simulink model "simulacao_sem_linearizar_prbs2"  (R2017a)
settings: Solver=VariableStepAuto  StartTime=0.0  StopTime=100  RelTol=1e-3
values from neighbouring files (symbols this model uses):
  a = -9128    [prepare_y_prbs.m]
undefined symbols (not defined in the file or in its folder): g, m
libraries: simulink x1
settings Model: Creator=Mateus  LastModifiedBy=Vicente

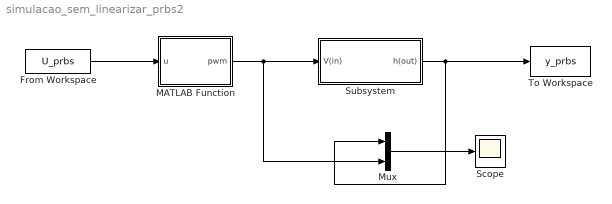
== system simulacao_sem_linearizar_prbs2 ==
  From Workspace : FromWorkspace  VariableName=U_prbs  SampleTime=0.05  Interpolate=off  OutputAfterFinalValue=Setting to zero
  MATLAB Function : MATLAB Function  TreatAsAtomicUnit=on
  Mux : Mux  Inputs=2
  Scope : Scope
  Subsystem : Subsystem
  To Workspace : ToWorkspace  VariableName=y_prbs  SaveFormat=Timeseries  SampleTime=0.05
  wires:
  From Workspace/1 -> MATLAB Function/1(u)
  MATLAB Function/1(pwm) -> Mux/2, Subsystem/1(V(in))
  Subsystem/1(h(out)) -> Mux/1, To Workspace/1
  Mux/1 -> Scope/1

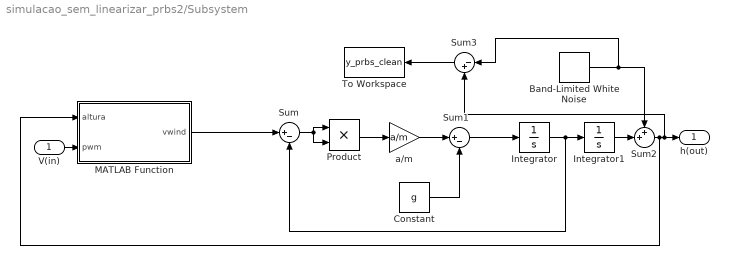
== system simulacao_sem_linearizar_prbs2/Subsystem ==
  V(in) : Inport
  Band-Limited White Noise : simulink/Sources/Band-Limited White Noise  Cov=[0.02]  Ts=0.1  seed=[23341]
  Constant : Constant  Value=g
  Integrator : Integrator
  Integrator1 : Integrator  InitialCondition=30
  MATLAB Function : MATLAB Function  TreatAsAtomicUnit=on
  Product : Product
  Sum : Sum  Inputs=|+-
  Sum1 : Sum  Inputs=|+-
  Sum2 : Sum  Inputs=++|
  Sum3 : Sum  Inputs=|-+
  To Workspace : ToWorkspace  VariableName=y_prbs_clean  SaveFormat=Timeseries  SampleTime=-1
  a/m : Gain  Gain=a/m
  h(out) : Outport
  wires:
  Sum2/1 -> Sum3/2, h(out)/1, MATLAB Function/1(altura)
  MATLAB Function/1(vwind) -> Sum/1
  Band-Limited White Noise/1 -> Sum3/1, Sum2/1
  Sum/1 -> Product/1, Product/2
  a/m/1 -> Sum1/1
  V(in)/1 -> MATLAB Function/2(pwm)
  Constant/1 -> Sum1/2
  Sum1/1 -> Integrator/1
  Product/1 -> a/m/1
  Integrator1/1 -> Sum2/2
  Integrator/1 -> Sum/2, Integrator1/1
  Sum3/1 -> To Workspace/1

== matlab function simulacao_sem_linearizar_prbs2/MATLAB Function ==
  data: u input; pwm output
function pwm = fcn(u)
if u==1
    pwm=26;
else
    pwm=64;
end

== matlab function simulacao_sem_linearizar_prbs2/Subsystem/MATLAB Function ==
  data: altura input; vwind output; pwm input
function vwind = fittedmodel(altura,pwm)

       p00 =       18.79;
       p10 =      -0.571;
       p01 =      0.2565;
       p20 =      0.0136;
       p11 =   -0.005502;
       p02 =  -0.0005601;
       p30 =   -0.000113;
       p21 =   4.503e-05;
       p12 =   5.745e-06;
       p03 =   3.291e-07;
       
       x=altura;
       y=pwm;

vwind= p00 + p10*x + p01*y + p20*x^2 + p11*x*y + p02*y^2 + p30*x^3 + p21*x^2*y + p12*x*y^2 + p03*y^3;
if vwind <0 
    vwind=0;
end

end
